simulink model "HydroEye_6DOF_HITL"  (R2024b)
settings: Solver=VariableStepAuto  StartTime=0.0  StopTime=1200  RelTol=1e-3
undefined symbols (not defined in the file): alpha_vec_Cn0, b, b_ref, beta_vec_Cn0, c, CD_flaps, CDo_CD_elev, cg, CL_flaps, Clbeta, Clda, CLo_CL_elev, Clo_Cl_rudder, Clp, Clr, Cm0, Cm_flaps, Cmda, Cmde, Cmo_Cm_elev, Cmq, Cn0, Cnda, Cno_Cn_rudder, Cnp, Cnr, contact, control, cp, CX0, CXda, CXde, CYbeta, CYda, Cyo_Cy_rudder, CZ0, CZda, CZde, d_ref, Earth, F, fractalcoef, Light, m_to_mm, mass, MIL, ms_to_cms, Payload, ref_height, ref_lat, ref_lon, SampleTime, uT_to_gauss, WGS84
libraries: uavmavlinklib x7, simulink_extras x4, aerolibwind2 x3, aerolibatmos2 x2, aerolibasang x2, px4MAVLinkBridgelib x2, shared6dof x1, aerolibadyn x1, simulink x1, aerolibtransform2 x1, sensorgpslib x1, robotcorelib x1
(part 1 of 2)
settings Model: Creator=01  LastModifiedBy=01
settings OptimizationCC: ReuseModelBlockBuffer=off
settings RTWCC: GPUComputeCapability=3.5

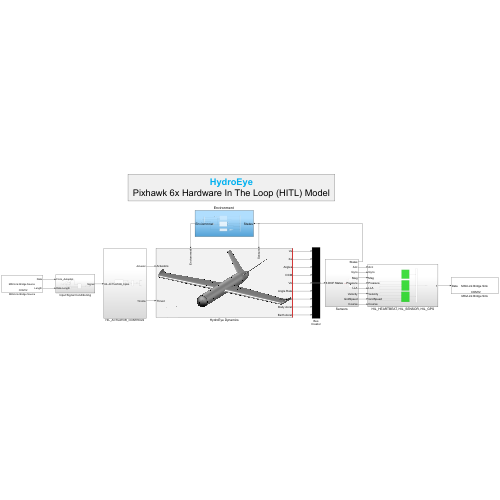
[thumbnail: Simulink's stored preview of the top-level diagram]
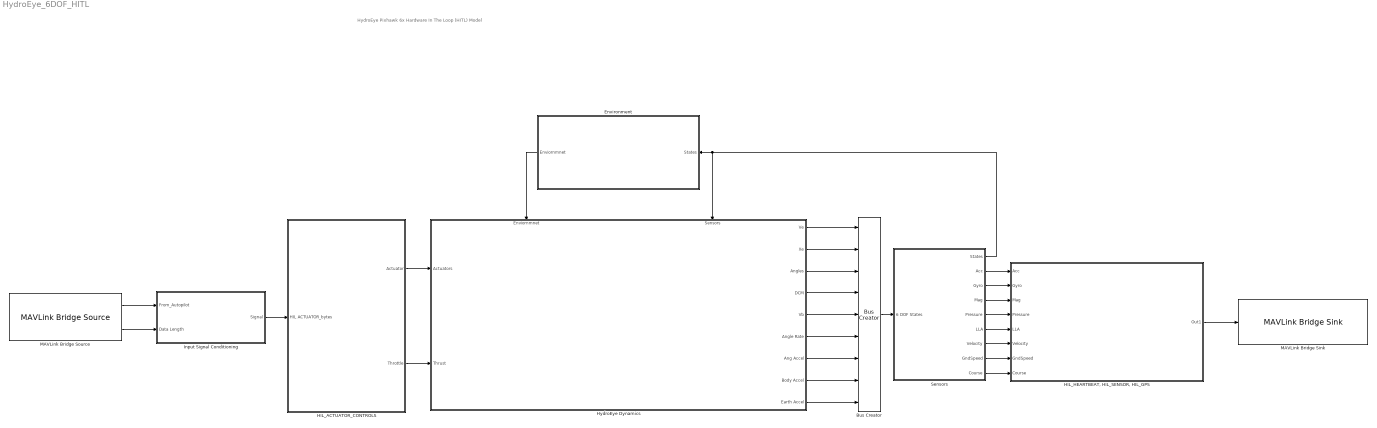
== system HydroEye_6DOF_HITL ==
  note: HydroEye
      | Pixhawk 6x Hardware In The Loop (HITL) Model
  Bus Creator : BusCreator  Inputs=9
  "Environment " : Subsystem
      settings: LibrarySourceBlock=|
      | aeroblk_lib_HL20/HL20
      | Airframe/Environment Models
  HIL_ACTUATOR_CONTROLS : Subsystem
  "HIL_HEARTBEAT, HIL_SENSOR, HIL_GPS" : Subsystem
  HydroEye Dynamics : Subsystem
      settings: PortSchema="{\"entries\":[{\"content\":{\"sides\":[{\"content\":{\"connectorIds\":[\"In1\",\"In2\"]},\"type\":\"ConnectorPlacement.EquallySpacedRectSide\",\"uuid\":\"55fccbc5-ee7f-44af-8150-33bff5380d0a\"},{\"content\":{\"connectorIds\":[\"Out1\",\"Out2\",\"Out3\",\"Out4\",\"Out5\",\"Out6\",\"Out7\",\"Out8\",\"Out9\"],\"side\":\"RIGHT\"},\"type\":\"ConnectorPlacement.EquallySpacedRectSide\",\"uuid\":\"71396e1b-5d20-4c4e-8e08-515b892d20e7\"},{\"content\":{\"connectorIds\":[\"In3\",\"In4\"],\"side\":\"TOP\"},\"type\":\"ConnectorPlacement.EquallySpacedRectSide\",\"uuid\":\"0174f631-e350-4c9f-98c1-67a3807d9144\"}]},\"type\":\"ConnectorPlacement.EquallySpacedConnector\",\"uuid\":\"de3a6adf-aa37-4a7c-9368-465ba59bc2f3\"}],\"packageUris\":[\"http://schema.mathworks.com/mf0/Connector/R2020b\"],\"version\":\"1.0\"}"
      mask Display: image('s.PNG');
  Input Signal Conditioning : Subsystem
  MAVLink Bridge Sink : px4MAVLinkBridgelib/MAVLink Bridge Sink  PixhawkSerialPorttemp=Specify manually  PixhawkSerialPortManually=COM12  FieldTable={ 'UDP', '127.0.0.1', '14550' }
  MAVLink Bridge Source : px4MAVLinkBridgelib/MAVLink Bridge Source  PixhawkSerialPorttemp=Specify manually  PixhawkSerialPortManually=COM12  dataLength=MAVLink_Input_Read_Size  FieldTable={ 'UDP', '127.0.0.1', '14550' }  SampleTime=SampleTime
  Sensors : Subsystem
  wires:
  Sensors/1(States) -> HydroEye Dynamics/4(Sensors), "Environment "/1(States)
  Bus Creator/1 -> Sensors/1(6 DOF States)
  HydroEye Dynamics/2(Xe) -> Bus Creator/2
  "Environment "/1(Enviornmnet) -> HydroEye Dynamics/3(Enviornmnet)
  HydroEye Dynamics/1(Ve) -> Bus Creator/1
  HydroEye Dynamics/3(Angles) -> Bus Creator/3
  HydroEye Dynamics/4(DCM) -> Bus Creator/4
  HydroEye Dynamics/5(Vb) -> Bus Creator/5
  HydroEye Dynamics/6(Angle Rate) -> Bus Creator/6
  HydroEye Dynamics/7(Ang Accel) -> Bus Creator/7
  HydroEye Dynamics/8(Body Accel) -> Bus Creator/8
  HydroEye Dynamics/9(Earth Accel) -> Bus Creator/9
  MAVLink Bridge Source/1 -> Input Signal Conditioning/1(From_Autopilot)
  MAVLink Bridge Source/2 -> Input Signal Conditioning/2(Data Length)
  HIL_ACTUATOR_CONTROLS/1(Actuator) -> HydroEye Dynamics/1(Actuators)
  Sensors/2(Acc) -> "HIL_HEARTBEAT, HIL_SENSOR, HIL_GPS"/1(Acc)
  Sensors/3(Gyro) -> "HIL_HEARTBEAT, HIL_SENSOR, HIL_GPS"/2(Gyro)
  Sensors/4(Mag) -> "HIL_HEARTBEAT, HIL_SENSOR, HIL_GPS"/3(Mag)
  Sensors/5(Pressure) -> "HIL_HEARTBEAT, HIL_SENSOR, HIL_GPS"/4(Pressure)
  Sensors/6(LLA) -> "HIL_HEARTBEAT, HIL_SENSOR, HIL_GPS"/5(LLA)
  Sensors/7(Velocity) -> "HIL_HEARTBEAT, HIL_SENSOR, HIL_GPS"/6(Velocity)
  Sensors/8(GndSpeed) -> "HIL_HEARTBEAT, HIL_SENSOR, HIL_GPS"/7(GndSpeed)
  Sensors/9(Course) -> "HIL_HEARTBEAT, HIL_SENSOR, HIL_GPS"/8(Course)
  "HIL_HEARTBEAT, HIL_SENSOR, HIL_GPS"/1(Out1) -> MAVLink Bridge Sink/1
  Input Signal Conditioning/1(Signal) -> HIL_ACTUATOR_CONTROLS/1(HIL ACTUATOR_bytes)
  HIL_ACTUATOR_CONTROLS/2(Throttle) -> HydroEye Dynamics/2(Thrust)

== system HydroEye_6DOF_HITL/Environment  ==
  States : Inport
  Bus Creator : BusCreator  Inputs=5
  Bus Selector : BusSelector  OutputSignals=Raw States.Ve,Raw States.DCM,LLA
  COESA Atmosphere Model : aerolibatmos2/COESA Atmosphere Model  units=Metric (MKS)  spec=1976 COESA-extended U.S. Standard Atmosphere  model=Profile  profile_var=High temperature  profile_percent=10%  profile_alt=5 km (16404 ft)  envelope_var=High temperature  envelope_percent=1%  action=None
      settings: LibrarySourceBlock=|
      | aeroblk_lib_HL20/HL20
      | Airframe/Environment Models/COESA Atmosphere Model
  Dot Product : DotProduct  Commented=on  SaturateOnIntegerOverflow=on  InputSameDT=off  OutDataTypeStr=Inherit: Inherit via internal rule
  Gravity in Earth Axes : Gain  Gain=[ 0 0 1]  SaturateOnIntegerOverflow=on  OutDataTypeStr=Inherit: Same as input  ParamDataTypeStr=Inherit: Same as input
  Selector : Selector  InputPortWidth=3  IndexOptions=Index vector (dialog)  Indices=3  OutputSizes=1
  Terminator : Terminator
  Terminator1 : Terminator
  V : Math  Commented=on  Operator=sqrt  SignedPower=on
  "WGS84 Gravity Model  " : GravityWGS84  action=None
  Wind : Subsystem  Commented=on
  Enviornmnet : Outport
  wires:
  V/1 -> Wind/1(Airspeed)
  "WGS84 Gravity Model  "/1 -> Gravity in Earth Axes/1
  COESA Atmosphere Model/1 -> Terminator/1
  COESA Atmosphere Model/3 -> Terminator1/1
  COESA Atmosphere Model/2 -> Bus Creator/3
  COESA Atmosphere Model/4 -> Bus Creator/4  "rho"
  Selector/1 -> Wind/2(Altitude), COESA Atmosphere Model/1
  Dot Product/1 -> V/1
  Wind/2(p,q,r wind) -> Bus Creator/2  "p,q,r wind"
  Wind/1(u,v,w wind) -> Bus Creator/1  "u,v,w wind"
  Gravity in Earth Axes/1 -> Bus Creator/5  "gravity acceleration"
  States/1 -> Bus Selector/1
  Bus Selector/2 -> Wind/3(DCM)  "<DCM>"
  Bus Selector/1 -> Dot Product/1, Dot Product/2  "<Ve>"
  Bus Selector/3 -> "WGS84 Gravity Model  "/1, Selector/1  "<LLA>"
  Bus Creator/1 -> Enviornmnet/1  "Environment"

== system HydroEye_6DOF_HITL/HIL_ACTUATOR_CONTROLS ==
  HIL ACTUATOR_bytes : Inport
  Bus Selector : BusSelector  OutputSignals=Payload.controls
  Data Type Conversion : DataTypeConversion  OutDataTypeStr=double  SaturateOnIntegerOverflow=off  RndMeth=Floor
  MAVLink Deserializer : uavmavlinklib/MAVLink Deserializer  dialectSource=Select from standard MAVLink dialects  dialect=common.xml  dialectCustom=common.xml  version=2  messageType=HIL_ACTUATOR_CONTROLS  inputDataLength=off  SystemIDFilter=off  systemID=1  ComponentIDFilter=off  componentID=1  queueMsg=off  queueMsgSize=50  dropNum=off
  Saturation : Saturate  UpperLimit=1  LowerLimit=0
  Selector1 : Selector  InputPortWidth=16  IndexOptions=Index vector (dialog)  Indices=[1:4]  OutputSizes=1
  Terminator : Terminator
  Actuator : Outport
  Throttle : Outport  Port=2
  wires:
  Data Type Conversion/1 -> Selector1/1
  MAVLink Deserializer/1 -> Terminator/1
  MAVLink Deserializer/2 -> Bus Selector/1
  Bus Selector/1 -> Data Type Conversion/1  "<controls>"
  HIL ACTUATOR_bytes/1 -> MAVLink Deserializer/1
  Selector1/1 -> Saturation/1  "Controls"
  Saturation/1 -> Throttle/1, Actuator/1

== system HydroEye_6DOF_HITL/HIL_HEARTBEAT, HIL_SENSOR, HIL_GPS ==
  Acc : Inport
  Gyro : Inport  Port=2
  Mag : Inport  Port=3
  Pressure : Inport  Port=4
  LLA : Inport  Port=5
  Velocity : Inport  Port=6
  GndSpeed : Inport  Port=7
  Course : Inport  Port=8
  HIL_GPS : Subsystem
  HIL_SENSOR : Subsystem
  Mux : Mux  Inputs=3
  Send Heartbeat : Subsystem
  Out1 : Outport
  wires:
  Send Heartbeat/1(HEARTBEAT_bytes) -> Mux/1
  Velocity/1 -> HIL_GPS/2(Velocity)
  HIL_GPS/1(HIL_GPS_bytes) -> Mux/3
  HIL_SENSOR/1(HIL_SENSOR_bytes) -> Mux/2
  GndSpeed/1 -> HIL_GPS/3(GndSpeed)
  LLA/1 -> HIL_GPS/1(LLA)
  Mag/1 -> HIL_SENSOR/3(Mag)
  Mux/1 -> Out1/1
  Pressure/1 -> HIL_SENSOR/4(Pressure)
  Course/1 -> HIL_GPS/4(Course)
  Gyro/1 -> HIL_SENSOR/2(Gyro)
  Acc/1 -> HIL_SENSOR/1(Acc)

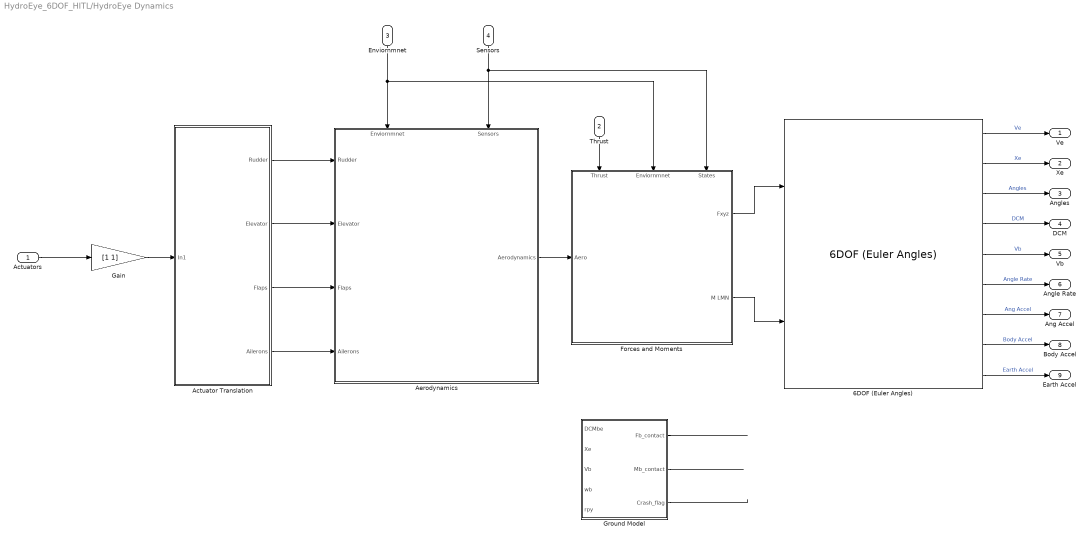
== system HydroEye_6DOF_HITL/HydroEye Dynamics ==
  Actuators : Inport
  Thrust : Inport  Port=2
  Enviornmnet : Inport  Port=3
  Sensors : Inport  Port=4
  6DOF (Euler Angles) : shared6dof/6DOF (Euler Angles)  units=Metric (MKS)  mtype=Fixed  rep=Euler Angles  xme_0=init.pos  Vm_0=init.v  eul_0=init.angles  pm_0=init.angRates  mass_0=mass  mass_e=0.5  mass_f=2.0  inertia=I  inertia_e=eye(3)  inertia_f=2*eye(3)  k_quat=1.0  vre_flag=on  abi_flag=on  aMode=aMode  xme_statename=''  Vm_statename=''  eul_statename=''  quat_statename=''  pm_statename=''  mass_statename=''
      settings: LibrarySourceBlock=|
      | aeroblk_lib_HL20/HL20
      | Airframe/6DOF (Euler Angles)
  Actuator Translation : Subsystem
  Aerodynamics : Subsystem
      settings: PortSchema="{\"entries\":[{\"content\":{\"sides\":[{\"content\":{\"connectorIds\":[\"In1\",\"In2\"]},\"type\":\"ConnectorPlacement.EquallySpacedRectSide\",\"uuid\":\"6872a9e6-04cc-43fe-8307-2d3d33caa71d\"},{\"content\":{\"side\":\"RIGHT\"},\"type\":\"ConnectorPlacement.EquallySpacedRectSide\",\"uuid\":\"de5f8d1c-5c0e-46cb-94c5-3e4cce4cf93c\"},{\"content\":{\"connectorIds\":[\"In3\",\"In4\",\"In5\",\"In6\"],\"side\":\"TOP\"},\"type\":\"ConnectorPlacement.EquallySpacedRectSide\",\"uuid\":\"d9dd98e0-8ff1-4387-90e5-0ec057a718ca\"},{\"content\":{\"connectorIds\":[\"Out1\"],\"side\":\"BOTTOM\"},\"type\":\"ConnectorPlacement.EquallySpacedRectSide\",\"uuid\":\"12421dae-0177-4f1a-9b31-64f8981b692b\"}]},\"type\":\"ConnectorPlacement.EquallySpacedConnector\",\"uuid\":\"9e39648a-6fb6-4479-b0ac-1c0f654141e6\"}],\"packageUris\":[\"http://schema.mathworks.com/mf0/Connector/R2020b\"],\"version\":\"1.0\"}"
  Forces and Moments : Subsystem
      settings: PortSchema="{\"entries\":[{\"content\":{\"sides\":[{\"content\":{\"connectorIds\":[\"In1\"]},\"type\":\"ConnectorPlacement.EquallySpacedRectSide\",\"uuid\":\"3fce203a-ae0b-4bce-a87b-30de4173aaf5\"},{\"content\":{\"connectorIds\":[\"Out1\",\"Out2\"],\"side\":\"RIGHT\"},\"type\":\"ConnectorPlacement.EquallySpacedRectSide\",\"uuid\":\"d2fe57eb-25a4-4a3f-81a0-5ad8de127e30\"},{\"content\":{\"connectorIds\":[\"In2\",\"In3\",\"In4\"],\"side\":\"TOP\"},\"type\":\"ConnectorPlacement.EquallySpacedRectSide\",\"uuid\":\"a48e6f39-78f9-49f0-a87f-61fc55168fed\"}]},\"type\":\"ConnectorPlacement.EquallySpacedConnector\",\"uuid\":\"9bf99150-9e27-4a02-9f3a-86824a85a991\"}],\"packageUris\":[\"http://schema.mathworks.com/mf0/Connector/R2020b\"],\"version\":\"1.0\"}"
      settings: LibrarySourceBlock=|
      | aeroblk_lib_HL20/HL20
      | Airframe/Forces and Moments
  Gain : Gain  Gain=[1 1]
  Ground Model : Subsystem
  Ve : Outport
  Xe : Outport  Port=2
  Angles : Outport  Port=3
  DCM : Outport  Port=4
  Vb : Outport  Port=5
  Angle Rate : Outport  Port=6
  Ang Accel : Outport  Port=7
  Body Accel : Outport  Port=8
  Earth Accel : Outport  Port=9
  wires:
  Forces and Moments/1(Fxyz) -> 6DOF (Euler Angles)/1
  Sensors/1 -> Forces and Moments/4(States), Aerodynamics/2(Sensors)
  Enviornmnet/1 -> Forces and Moments/3(Enviornmnet), Aerodynamics/1(Enviornmnet)
  Forces and Moments/2(M LMN) -> 6DOF (Euler Angles)/2
  Actuators/1 -> Gain/1
  6DOF (Euler Angles)/4 -> DCM/1  "DCM"
  6DOF (Euler Angles)/2 -> Xe/1  "Xe"
  6DOF (Euler Angles)/1 -> Ve/1  "Ve"
  6DOF (Euler Angles)/3 -> Angles/1  "Angles"
  6DOF (Euler Angles)/6 -> Angle Rate/1  "Angle Rate"
  6DOF (Euler Angles)/8 -> Body Accel/1  "Body Accel"
  6DOF (Euler Angles)/5 -> Vb/1  "Vb"
  6DOF (Euler Angles)/9 -> Earth Accel/1  "Earth Accel"
  6DOF (Euler Angles)/7 -> Ang Accel/1  "Ang Accel"
  Thrust/1 -> Forces and Moments/2(Thrust)
  Ground Model/3(Crash_flag) -> ?
  Ground Model/1(Fb_contact) -> ?
  Ground Model/2(Mb_contact) -> ?
  Aerodynamics/1("Aerodynamics ") -> Forces and Moments/1(Aero)
  Gain/1 -> Actuator Translation/1(In1)
  Actuator Translation/1(Rudder) -> Aerodynamics/3(Rudder)
  Actuator Translation/2(Elevator) -> Aerodynamics/4(Elevator)
  Actuator Translation/3(Flaps) -> Aerodynamics/5(Flaps)
  Actuator Translation/4(Ailerons) -> Aerodynamics/6(Ailerons)

== system HydroEye_6DOF_HITL/Input Signal Conditioning ==
  From_Autopilot : Inport
  Data Length : Inport  Port=2
  Constant : Constant
  Constant1 : Constant  Value=0  OutDataTypeStr=uint8  SampleTime=-1
  Data Type Conversion : DataTypeConversion  OutDataTypeStr=double  SaturateOnIntegerOverflow=off  RndMeth=Floor
  Mux1 : Mux  Inputs=2
  Reshape : Reshape
  Selector : Selector  InputPortWidth=MAVLink_Input_Read_Size  IndexOptions=Starting and ending indices (port)  Indices=[1 3]  OutputSizes=1
  Switch : Switch  Criteria=u2 > Threshold  SaturateOnIntegerOverflow=off  InputSameDT=off
  Signal : Outport
  wires:
  Reshape/1 -> Signal/1
  Mux1/1 -> Selector/2
  Data Length/1 -> Data Type Conversion/1
  Constant/1 -> Mux1/1
  Selector/1 -> Switch/1
  From_Autopilot/1 -> Selector/1
  Constant1/1 -> Switch/3
  Switch/1 -> Reshape/1
  Data Type Conversion/1 -> Switch/2, Mux1/2

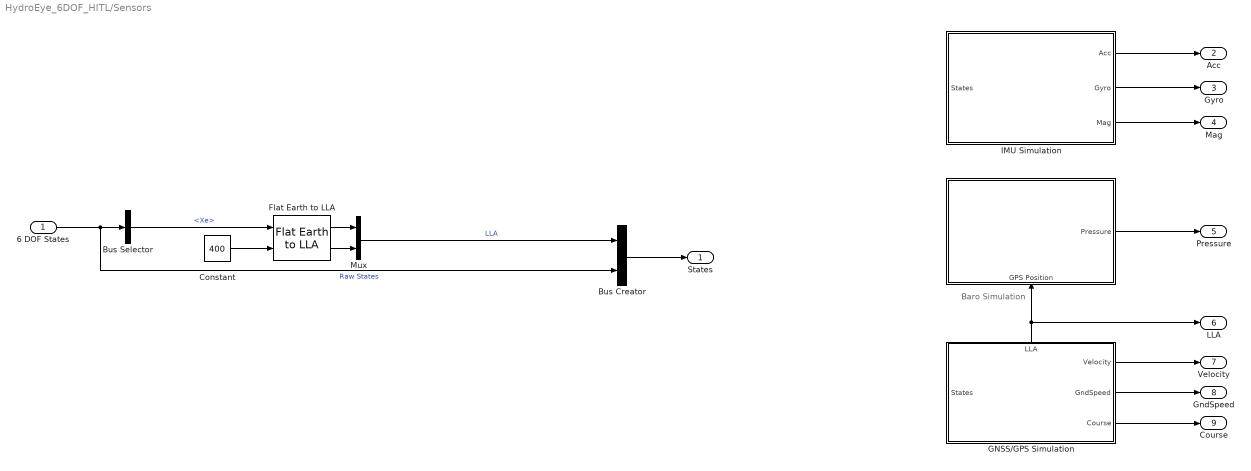
== system HydroEye_6DOF_HITL/Sensors ==
  note: Baro Simulation
  6 DOF States : Inport
  " " : Subsystem
      settings: PortSchema="{\"entries\":[{\"content\":{\"sides\":[{\"content\":{\"connectorIds\":[]},\"type\":\"ConnectorPlacement.EquallySpacedRectSide\",\"uuid\":\"7ecc8b21-8f8f-4144-826a-6b68e30dbf7d\"},{\"content\":{\"connectorIds\":[\"Out1\"],\"side\":\"RIGHT\"},\"type\":\"ConnectorPlacement.EquallySpacedRectSide\",\"uuid\":\"81a1dd55-8330-4386-9921-36c0eb60d526\"},{\"content\":{\"connectorIds\":[],\"side\":\"TOP\"},\"type\":\"ConnectorPlacement.EquallySpacedRectSide\",\"uuid\":\"b99caff5-b40d-407d-b30e-35210c1aee1d\"},{\"content\":{\"connectorIds\":[\"In1\"],\"side\":\"BOTTOM\"},\"type\":\"ConnectorPlacement.EquallySpacedRectSide\",\"uuid\":\"18bfda3d-4fab-4e61-9ebc-e384e51de306\"}]},\"type\":\"ConnectorPlacement.EquallySpacedConnector\",\"uuid\":\"17ab4e96-b761-4c62-a0bb-ab626dac3eaa\"}],\"packageUris\":[\"http://schema.mathworks.com/mf0/Connector/R2020b\"],\"version\":\"1.0\"}"
  Bus Creator : BusCreator  Inputs=2
  Bus Selector : BusSelector  OutputSignals=Xe
  Constant : Constant  Value=400
  Flat Earth to LLA : aerolibtransform2/Flat Earth to LLA  units=Metric (MKS)  ptype=Earth (WGS84)  F=1/298.257223563  R=6378137  refPosPort=off  LL0=[ 24 46 ]  psi=0
  GNSS/GPS Simulation : Subsystem
      settings: PortSchema="{\"entries\":[{\"content\":{\"sides\":[{\"content\":{\"connectorIds\":[\"In1\"]},\"type\":\"ConnectorPlacement.EquallySpacedRectSide\",\"uuid\":\"4934e8ff-5d4b-4e11-968d-c23bd62383a0\"},{\"content\":{\"connectorIds\":[\"Out1\",\"Out2\",\"Out3\"],\"side\":\"RIGHT\"},\"type\":\"ConnectorPlacement.EquallySpacedRectSide\",\"uuid\":\"9ec8bc0a-2d3c-4dca-835c-010ac29b6ebc\"},{\"content\":{\"connectorIds\":[\"Out4\"],\"side\":\"TOP\"},\"type\":\"ConnectorPlacement.EquallySpacedRectSide\",\"uuid\":\"04f09eb4-1bd9-450e-b951-47054bdd92ad\"}]},\"type\":\"ConnectorPlacement.EquallySpacedConnector\",\"uuid\":\"9a5920cf-a58d-4c98-839b-fbac94edbe7e\"}],\"packageUris\":[\"http://schema.mathworks.com/mf0/Connector/R2020b\"],\"version\":\"1.0\"}"
  IMU Simulation : Subsystem
  Mux : Mux  Inputs=2
  States : Outport
  Acc : Outport  Port=2
  Gyro : Outport  Port=3
  Mag : Outport  Port=4
  Pressure : Outport  Port=5
  LLA : Outport  Port=6
  Velocity : Outport  Port=7
  GndSpeed : Outport  Port=8
  Course : Outport  Port=9
  wires:
  6 DOF States/1 -> Bus Creator/2, Bus Selector/1  "Raw States"
  Bus Selector/1 -> Flat Earth to LLA/1  "<Xe>"
  Flat Earth to LLA/2 -> Mux/2
  Flat Earth to LLA/1 -> Mux/1
  Mux/1 -> Bus Creator/1  "LLA"
  Bus Creator/1 -> States/1
  Constant/1 -> Flat Earth to LLA/2
  GNSS/GPS Simulation/1(Velocity) -> Velocity/1
  " "/1(Pressure) -> Pressure/1
  ? -> IMU Simulation/1(States), GNSS/GPS Simulation/1(States)
  IMU Simulation/3(Mag) -> Mag/1
  GNSS/GPS Simulation/3(Course) -> Course/1
  GNSS/GPS Simulation/2(GndSpeed) -> GndSpeed/1
  GNSS/GPS Simulation/4(LLA) -> LLA/1, " "/1(GPS Position)
  IMU Simulation/2(Gyro) -> Gyro/1
  IMU Simulation/1(Acc) -> Acc/1

== system HydroEye_6DOF_HITL/Environment /Wind ==
  Airspeed : Inport  Unit=m/s
  Altitude : Inport  Port=2  Unit=m
  DCM : Inport  Port=3
  Discrete Wind Gust Model - On : aerolibwind2/Discrete Wind Gust Model  units=Metric (MKS)  Gx=on  Gy=on  Gz=on  t_0=20  d_m=[120 120 80]  v_m=[3.5 3.0 3.0]
      settings: LibrarySourceBlock=|
      | aeroblk_lib_HL20/HL20
      | Airframe/Environment Models/Wind Models/Discrete Wind Gust Model - On
  Dryden Wind Turbulence Model (Continuous (+q -r)) : aerolibwind2/Dryden Wind Turbulence Model  (Continuous (+q -r))  units=Metric (MKS)  spec=MIL-F-8785C  model=Continuous Dryden (+q -r)  W20=5  Wdeg=0  TurbProb=10^-2 - Light  L_high=533.4  Wingspan=4  ts=0.1  Seed=[23341 23342 23343 23344]  T_on=on
      settings: LibrarySourceBlock=|
      | aeroblk_lib_HL20/HL20
      | Airframe/Environment Models/Wind Models/Dryden Wind Turbulence Model
      | (Continuous (+q -r))
  Sum : Sum  Inputs=+++  InputSameDT=on  SaturateOnIntegerOverflow=on  OutDataTypeStr=Inherit: Same as first input
  Wind Shear Model : aerolibwind2/Wind Shear Model  units=Metric (MKS)  phase=Category C - Terminal Flight Phase  W_20=1  Wdeg=0
      settings: LibrarySourceBlock=|
      | aeroblk_lib_HL20/HL20
      | Airframe/Environment Models/Wind Models/Wind Shear Model
  u,v,w wind : Outport  Unit=m/s  VectorParamsAs1DForOutWhenUnconnected=off
  p,q,r wind : Outport  Port=2  Unit=rad/s  VectorParamsAs1DForOutWhenUnconnected=off
  wires:
  Altitude/1 -> Wind Shear Model/1, Dryden Wind Turbulence Model (Continuous (+q -r))/1
  Dryden Wind Turbulence Model (Continuous (+q -r))/2 -> p,q,r wind/1
  Airspeed/1 -> Discrete Wind Gust Model - On/1, Dryden Wind Turbulence Model (Continuous (+q -r))/2
  DCM/1 -> Wind Shear Model/2, Dryden Wind Turbulence Model (Continuous (+q -r))/3
  Sum/1 -> u,v,w wind/1
  Discrete Wind Gust Model - On/1 -> Sum/3
  Dryden Wind Turbulence Model (Continuous (+q -r))/1 -> Sum/2
  Wind Shear Model/1 -> Sum/1

== system HydroEye_6DOF_HITL/HIL_HEARTBEAT, HIL_SENSOR, HIL_GPS/HIL_GPS ==
  LLA : Inport
  Velocity : Inport  Port=2
  GndSpeed : Inport  Port=3
  Course : Inport  Port=4
  HIL_GPS Subsystem : Subsystem
  MAVLink Serializer3 : uavmavlinklib/MAVLink Serializer  dialectSource=Select from standard MAVLink dialects  dialect=common.xml  dialectCustom=common.xml  version=2  messageType=HIL_GPS
  Rate Transition : RateTransition  OutPortSampleTime=SampleTime
  Terminator2 : Terminator
  HIL_GPS_bytes : Outport
  wires:
  HIL_GPS Subsystem/1(Out1) -> Rate Transition/1
  Course/1 -> HIL_GPS Subsystem/4(Course)
  MAVLink Serializer3/2 -> Terminator2/1
  LLA/1 -> HIL_GPS Subsystem/1(LLA)
  GndSpeed/1 -> HIL_GPS Subsystem/3(GndSpeed)
  MAVLink Serializer3/1 -> HIL_GPS_bytes/1
  Velocity/1 -> HIL_GPS Subsystem/2(Velocity)
  Rate Transition/1 -> MAVLink Serializer3/1

== system HydroEye_6DOF_HITL/HIL_HEARTBEAT, HIL_SENSOR, HIL_GPS/HIL_SENSOR ==
  Acc : Inport
  Gyro : Inport  Port=2
  Mag : Inport  Port=3
  Pressure : Inport  Port=4
  HIL_SENSOR Creation subsystem : Subsystem
  MAVLink Serializer1 : uavmavlinklib/MAVLink Serializer  dialectSource=Select from standard MAVLink dialects  dialect=common.xml  dialectCustom=common.xml  version=2  messageType=HIL_SENSOR
  Rate Transition : RateTransition  OutPortSampleTime=SampleTime
  Terminator : Terminator
  HIL_SENSOR_bytes : Outport
  wires:
  Pressure/1 -> HIL_SENSOR Creation subsystem/4(Pressure)
  Acc/1 -> HIL_SENSOR Creation subsystem/1(Acc)
  MAVLink Serializer1/2 -> Terminator/1
  MAVLink Serializer1/1 -> HIL_SENSOR_bytes/1
  Mag/1 -> HIL_SENSOR Creation subsystem/3(Mag)
  HIL_SENSOR Creation subsystem/1(HIL Sensor) -> Rate Transition/1
  Gyro/1 -> HIL_SENSOR Creation subsystem/2(Gyro)
  Rate Transition/1 -> MAVLink Serializer1/1

== system HydroEye_6DOF_HITL/HIL_HEARTBEAT, HIL_SENSOR, HIL_GPS/Send Heartbeat ==
  Bus Assignment : BusAssignment  AssignedSignals=Payload.autopilot,Payload.type
  Constant : Constant  SampleTime=-1
  Constant1 : Constant  Value=12  SampleTime=-1
  Data Type Conversion : DataTypeConversion  OutDataTypeStr=uint8  SaturateOnIntegerOverflow=off  RndMeth=Floor
  Data Type Conversion1 : DataTypeConversion  OutDataTypeStr=uint8  SaturateOnIntegerOverflow=off  RndMeth=Floor
  MAVLink Blank Message : uavmavlinklib/MAVLink Blank Message  dialectSource=Select from standard MAVLink dialects  dialect=common.xml  dialectCustom=common.xml  version=2  messageType=HEARTBEAT  SystemID=2  ComponentID=51  SampleTime=SampleTime
  MAVLink Serializer : uavmavlinklib/MAVLink Serializer  dialectSource=Select from standard MAVLink dialects  dialect=common.xml  dialectCustom=common.xml  version=2  messageType=HEARTBEAT
  Terminator4 : Terminator
  HEARTBEAT_bytes : Outport
  wires:
  Bus Assignment/1 -> MAVLink Serializer/1
  Constant/1 -> Data Type Conversion/1
  MAVLink Serializer/1 -> HEARTBEAT_bytes/1
  Data Type Conversion1/1 -> Bus Assignment/3
  Data Type Conversion/1 -> Bus Assignment/2
  MAVLink Serializer/2 -> Terminator4/1
  Constant1/1 -> Data Type Conversion1/1
  MAVLink Blank Message/1 -> Bus Assignment/1

== system HydroEye_6DOF_HITL/HydroEye Dynamics/Actuator Translation ==
  note: https://ardupilot.org/plane/docs/guide-vtail-plane.html#guide-vtail-plane
      |
      | Basically reversed ArduPilot's V-tail mixing, to translate to an elevator & rudder config, making us need less data.
      |
      | So the rudder commads in deg for each ruddervator is mixed as a percentage of elevator adn rudder deflection.
      |
      | The gain is a mixing percantage and it is IMPORTANT to update it when changing it in the parameters OR ELSE the translation will be wrong
  In1 : Inport
  Demux : Demux
  Gain : Gain  Gain=0.5
  Gain1 : Gain  Gain=0.5
  Sum : Sum  Inputs=|-+
  Sum1 : Sum  Inputs=|++
  Rudder : Outport
  Elevator : Outport  Port=2
  Flaps : Outport  Port=3
  Ailerons : Outport  Port=4
  wires:
  In1/1 -> Demux/1
  Demux/1 -> Gain/1  "Ruddervator Right"
  Demux/2 -> Gain1/1  "Ruddervator Left"
  Sum/1 -> Rudder/1
  Sum1/1 -> Elevator/1
  Gain/1 -> Sum1/1, Sum/1
  Gain1/1 -> Sum1/2, Sum/2
  Demux/3 -> Flaps/1  "Flaps"
  Demux/4 -> Ailerons/1  "Ailerons"

== system HydroEye_6DOF_HITL/HydroEye Dynamics/Aerodynamics ==
  note: Order is for stability input in aero forces block
  Enviornmnet : Inport
  Sensors : Inport  Port=2
  Rudder : Inport  Port=3
  Elevator : Inport  Port=4
  Flaps : Inport  Port=5
  Ailerons : Inport  Port=6
  Aero Coeff : Subsystem
  Aerodynamic Coefficients : Subsystem  Commented=on
      settings: LibrarySourceBlock=|
      | aeroblk_lib_HL20/HL20
      | Airframe/Aerodynamic
      | Coefficients
  Alpha,Beta,q : Subsystem
      settings: LibrarySourceBlock=|
      | aeroblk_lib_HL20/HL20
      | Airframe/Alpha,Beta,Mach
  Bus Creator : BusCreator  Inputs=2
  Demux : Demux  Outputs=2
  Mux : Mux  Inputs=6
  Radians to Degrees : simulink_extras/Transformations/Radians to Degrees
  Radians to Degrees1 : simulink_extras/Transformations/Radians to Degrees
  "Aerodynamics " : Outport
  wires:
  Sensors/1 -> Aero Coeff/7(Sensors), Alpha,Beta,q/2(Sensors)
  Enviornmnet/1 -> Alpha,Beta,q/1(Enviornmnet)
  Alpha,Beta,q/2(qbar) -> Bus Creator/2  "qbar"
  Mux/1 -> Bus Creator/1  "Aero Coeff"
  Alpha,Beta,q/1(Incid) -> Demux/1
  Aero Coeff/1(CD) -> Mux/1  "CD"
  Aero Coeff/2(CY) -> Mux/2  "CY"
  Aero Coeff/3(CL) -> Mux/3  "CL"
  Aero Coeff/4(Cl) -> Mux/4  "Cl"
  Aero Coeff/5(Cm) -> Mux/5  "Cm"
  Aero Coeff/6(Cn) -> Mux/6  "Cn"
  Radians to Degrees/1 -> Aero Coeff/1(Alpha)  "alpha"
  Radians to Degrees1/1 -> Aero Coeff/2(Beta)  "beta"
  Demux/2 -> Radians to Degrees1/1
  Demux/1 -> Radians to Degrees/1  "a rad"
  Bus Creator/1 -> "Aerodynamics "/1
  Rudder/1 -> Aero Coeff/3(Rudder)
  Elevator/1 -> Aero Coeff/4(Elevator)
  Flaps/1 -> Aero Coeff/5(Flaps)
  Ailerons/1 -> Aero Coeff/6(Ailerons)

== system HydroEye_6DOF_HITL/HydroEye Dynamics/Forces and Moments ==
  Aero : Inport
  Thrust : Inport  Port=2
  Enviornmnet : Inport  Port=3
  States : Inport  Port=4
  Aerodynamic Forces and Moments : aerolibadyn/Aerodynamic Forces and Moments   inputAxes=Stability  outputForceAxes=Body  outputMomentAxes=Body  S=Sref  b=b  cbar=c
      settings: LibrarySourceBlock=|
      | aeroblk_lib_HL20/HL20
      | Airframe/Forces and Moments/Aerodynamic
      | Forces and Moments
  Bus Selector : BusSelector  OutputSignals=gravity acceleration
  Bus Selector1 : BusSelector  OutputSignals=Raw States.DCM,Raw States.Vb
  Bus Selector2 : BusSelector  OutputSignals=Aero Coeff,qbar
  Gain1 : Gain  Gain=mass
  Matrix Multiply : Product  Multiplication=Matrix(*)
  Sum : Sum  Inputs=+++  InputSameDT=on  SaturateOnIntegerOverflow=on  OutDataTypeStr=Inherit: Same as first input
  center of gravity : Constant  Value=cg
  center of pressure : Constant  Value=cp
  Fxyz : Outport
  M LMN : Outport  Port=2
  wires:
  Sum/1 -> Fxyz/1
  center of gravity/1 -> Aerodynamic Forces and Moments/3
  center of pressure/1 -> Aerodynamic Forces and Moments/4
  Enviornmnet/1 -> Bus Selector/1
  States/1 -> Bus Selector1/1
  Matrix Multiply/1 -> Sum/3
  Bus Selector/1 -> Gain1/1  "<gravity acceleration>"
  Gain1/1 -> Matrix Multiply/2
  Bus Selector1/1 -> Matrix Multiply/1  "<DCM>"
  Thrust/1 -> Sum/1
  Aerodynamic Forces and Moments/1 -> Sum/2  "Faero"
  Aerodynamic Forces and Moments/2 -> M LMN/1
  Bus Selector1/2 -> Aerodynamic Forces and Moments/5  "<Vb>"
  Aero/1 -> Bus Selector2/1
  Bus Selector2/1 -> Aerodynamic Forces and Moments/1  "<Aero Coeff>"
  Bus Selector2/2 -> Aerodynamic Forces and Moments/2  "<qbar>"

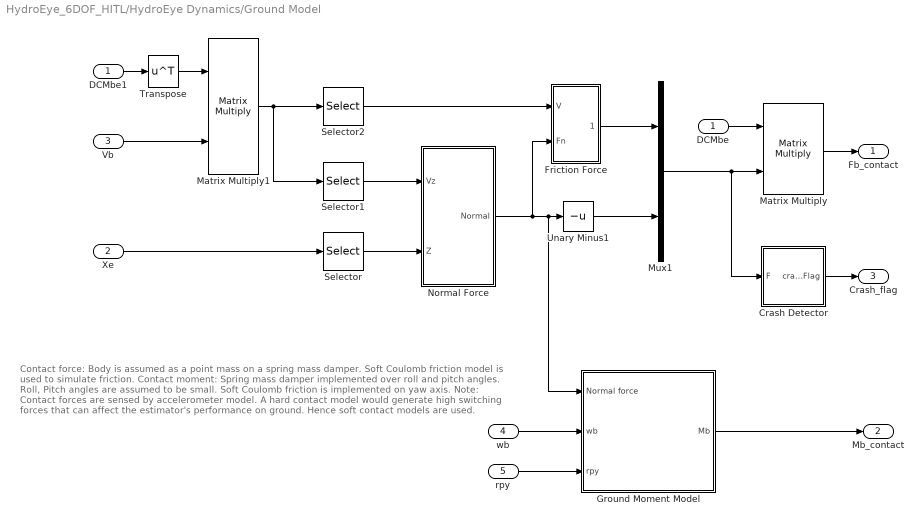
== system HydroEye_6DOF_HITL/HydroEye Dynamics/Ground Model ==
  note: Contact force:
      | Body is assumed as a point mass on a spring mass damper. Soft Coulomb friction model is used to simulate friction.
      |
      | Contact moment:
      | Spring mass damper implemented over roll and pitch angles. Roll, Pitch angles are assumed to be small.
      | Soft Coulomb friction is implemented on yaw axis.
      |
      | Note:
      | Contact forces are sensed by accelerometer model. A hard contact model would generate high switching forces that can affect the estimator's performance on ground. Hence soft contact models are used.
  DCMbe : Inport
  Xe : Inport  Port=2
  Vb : Inport  Port=3
  wb : Inport  Port=4
  rpy : Inport  Port=5
  Crash Detector : Subsystem
  DCMbe1 : InportShadow
  Friction Force : Subsystem
  Ground Moment Model : Subsystem
  Matrix Multiply : Product  Multiplication=Matrix(*)
  Matrix Multiply1 : Product  Multiplication=Matrix(*)
  Mux1 : Mux  Inputs=2
  Normal Force : Subsystem
  Selector : Selector  InputPortWidth=3  IndexOptions=Index vector (dialog)  Indices=[3]  OutputSizes=1
  Selector1 : Selector  InputPortWidth=3  IndexOptions=Index vector (dialog)  Indices=[3]  OutputSizes=1
  Selector2 : Selector  InputPortWidth=3  IndexOptions=Index vector (dialog)  Indices=[1,2]  OutputSizes=1
  Transpose : Math  Operator=transpose
  Unary Minus1 : UnaryMinus
  Fb_contact : Outport
  Mb_contact : Outport  Port=2
  Crash_flag : Outport  Port=3
  wires:
  Crash Detector/1(crashFlag) -> Crash_flag/1
  Xe/1 -> Selector/1
  Selector1/1 -> Normal Force/1(Vz)
  Selector/1 -> Normal Force/2(Z)
  DCMbe/1 -> Matrix Multiply/1
  Matrix Multiply/1 -> Fb_contact/1
  Normal Force/1(Normal) -> Ground Moment Model/1(Normal force), Unary Minus1/1, Friction Force/2(Fn)
  Mux1/1 -> Crash Detector/1(F), Matrix Multiply/2
  Unary Minus1/1 -> Mux1/2
  Selector2/1 -> Friction Force/1(V)
  Friction Force/1(Friction) -> Mux1/1
  DCMbe1/1 -> Transpose/1
  Transpose/1 -> Matrix Multiply1/1
  Vb/1 -> Matrix Multiply1/2
  Matrix Multiply1/1 -> Selector1/1, Selector2/1
  wb/1 -> Ground Moment Model/2(wb)
  rpy/1 -> Ground Moment Model/3(rpy)
  Ground Moment Model/1(Mb) -> Mb_contact/1

== system HydroEye_6DOF_HITL/Sensors/  ==
  GPS Position : Inport
  Extract Altitude : Selector  InputPortWidth=3  IndexOptions=Index vector (dialog)  Indices=[3]  OutputSizes=1
  Gain1 : Gain  Gain=1/m_to_mm
  Gain2 : Gain  Gain=m_to_mm
  Lapse Rate Model : aerolibatmos2/ISA Atmosphere Model  useExtended=off  action=Warning  custom=on  viscosityOut=off  g=9.80665  gamma=1.4  R=287.0531  L=0.0065  h_trop=11000  h_strat=20000  rho0=1.225  P0=101325  T0=288.15  h0=0  S=110.4  Tref=273.15  muref=1.716e-5
  Random Number1 : RandomNumber  Variance=10000  Seed=10  SampleTime=SampleTime
  Sum1 : Sum  Inputs=|++
  Terminator : Terminator
  Terminator1 : Terminator
  Terminator2 : Terminator
  Pressure : Outport
  wires:
  Lapse Rate Model/2 -> Terminator1/1
  Lapse Rate Model/4 -> Terminator2/1
  Lapse Rate Model/1 -> Terminator/1
  Lapse Rate Model/3 -> Pressure/1
  Sum1/1 -> Gain1/1
  Gain2/1 -> Sum1/1
  Extract Altitude/1 -> Gain2/1
  Gain1/1 -> Lapse Rate Model/1
  GPS Position/1 -> Extract Altitude/1
  Random Number1/1 -> Sum1/2  "Pressure_noise"

== system HydroEye_6DOF_HITL/Sensors/GNSS//GPS Simulation ==
  States : Inport
  Bus Selector : BusSelector  OutputSignals=dx,dy,dz  OutputAsBus=on
  Bus Selector1 : BusSelector  OutputSignals=X,Y,Z  OutputAsBus=on
  GPS : sensorgpslib/GPS  DispRefFrame=NED  PositionInputFormat=Local  ReferenceLocation=[ref_lat ref_lon ref_height]  HorizontalPositionAccuracy=0.01  VerticalPositionAccuracy=0.01  VelocityAccuracy=0.01  DecayFactor=0.99  SeedDouble=67  SimulateUsing=Interpreted execution
  Reshape1 : Reshape  OutputDimensionality=Row vector (2-D)
  Reshape3 : Reshape  OutputDimensionality=Row vector (2-D)
  Velocity : Outport
  GndSpeed : Outport  Port=2
  Course : Outport  Port=3
  LLA : Outport  Port=4
  wires:
  Reshape3/1 -> GPS/1
  GPS/1 -> LLA/1  "lla"
  Bus Selector1/1 -> Reshape3/1
  Bus Selector/1 -> Reshape1/1
  Reshape1/1 -> GPS/2
  GPS/2 -> Velocity/1
  States/1 -> Bus Selector/1, Bus Selector1/1
  GPS/3 -> GndSpeed/1
  GPS/4 -> Course/1

== system HydroEye_6DOF_HITL/Sensors/IMU Simulation ==
  note: Note:
      | we need specific force (accelerometer output) in A-G form, but block gives G-A.
  States : Inport
  Bus Selector1 : BusSelector  OutputSignals=p,q,r  OutputAsBus=on
  Bus Selector2 : BusSelector  OutputSignals=yaw,pitch,roll  OutputAsBus=on
  Bus Selector3 : BusSelector  OutputSignals=ddx,ddy,ddz  OutputAsBus=on
  Coordinate Transformation Conversion1 : robotcorelib/Coordinate Transformation Conversion  InputRepresentation=Euler Angles  InputEulerSequence=ZYX  ShowTrVecInputPort=on  OutputRepresentation=Quaternion  OutputEulerSequence=ZYX  ShowTrVecOutputPort=on  SimulateUsing=Interpreted execution
  Gain : Gain  Gain=-1
  IMU1 : mspsensorlib/IMU  DispRefFrame=NED  TemperaturePort=off  Temperature=25  MagneticFieldPort=off  MagneticFieldNED=[21.5 1.16 43.1]  MagneticFieldENU=[ -2.4169, 27.5550, 16.0849 ]  SeedDouble=87254  SimulateUsing=Interpreted execution  AccelParamsMeasurementRange=Inf  AccelParamsResolution=0  AccelParamsConstantBias=[ 0, 0, 0 ]  AccelParamsAxesMisalignment=[ 0, 0, 0 ]  AccelParamsNoiseDensity=0.0003  AccelParamsBiasInstability=[ 0, 0, 0 ]  AccelParamsBiasInstabilityNumerator=fractalcoef().Numerator  AccelParamsBiasInstabilityDenominator=fractalcoef().Denominator  AccelParamsRandomWalk=[ 0, 0, 0 ]  AccelParamsNoiseType=double-sided  AccelParamsTemperatureBias=[ 0, 0, 0 ]  AccelParamsTemperatureScaleFactor=[ 0, 0, 0 ]  GyroParamsMeasurementRange=Inf  GyroParamsResolution=0  GyroParamsConstantBias=[ 0, 0, 0 ]  GyroParamsAxesMisalignment=[ 0, 0, 0 ]  GyroParamsAccelerationBias=0.0001  GyroParamsNoiseDensity=0.01  GyroParamsBiasInstability=[ 0, 0, 0 ]  GyroParamsBiasInstabilityNumerator=fractalcoef().Numerator  GyroParamsBiasInstabilityDenominator=fractalcoef().Denominator  GyroParamsRandomWalk=[ 0, 0, 0 ]  GyroParamsNoiseType=double-sided  GyroParamsTemperatureBias=[ 0, 0, 0 ]  GyroParamsTemperatureScaleFactor=[ 0, 0, 0 ]  MagParamsMeasurementRange=Inf  MagParamsResolution=0  MagParamsConstantBias=[ 0, 0, 0 ]  MagParamsAxesMisalignment=[ 0, 0, 0 ]  MagParamsNoiseDensity=0.0005  MagParamsBiasInstability=[ 0, 0, 0 ]  MagParamsBiasInstabilityNumerator=fractalcoef().Numerator  MagParamsBiasInstabilityDenominator=fractalcoef().Denominator  MagParamsRandomWalk=[ 0, 0, 0 ]  MagParamsNoiseType=double-sided  MagParamsTemperatureBias=[ 0, 0, 0 ]  MagParamsTemperatureScaleFactor=[ 0, 0, 0 ]
  Reshape : Reshape  OutputDimensionality=Row vector (2-D)
  Reshape2 : Reshape  OutputDimensionality=Row vector (2-D)
  Reshape3 : Reshape  OutputDimensionality=Row vector (2-D)
  Acc : Outport
  Gyro : Outport  Port=2
  Mag : Outport  Port=3
  wires:
  Coordinate Transformation Conversion1/1 -> Reshape3/1
  Reshape3/1 -> IMU1/3
  IMU1/3 -> Mag/1
  IMU1/2 -> Gyro/1
  Reshape/1 -> IMU1/1
  Bus Selector3/1 -> Reshape/1
  IMU1/1 -> Gain/1
  Bus Selector1/1 -> Reshape2/1
  Bus Selector2/1 -> Coordinate Transformation Conversion1/1
  Reshape2/1 -> IMU1/2
  States/1 -> Bus Selector1/1, Bus Selector2/1, Bus Selector3/1
  Gain/1 -> Acc/1  "acc"

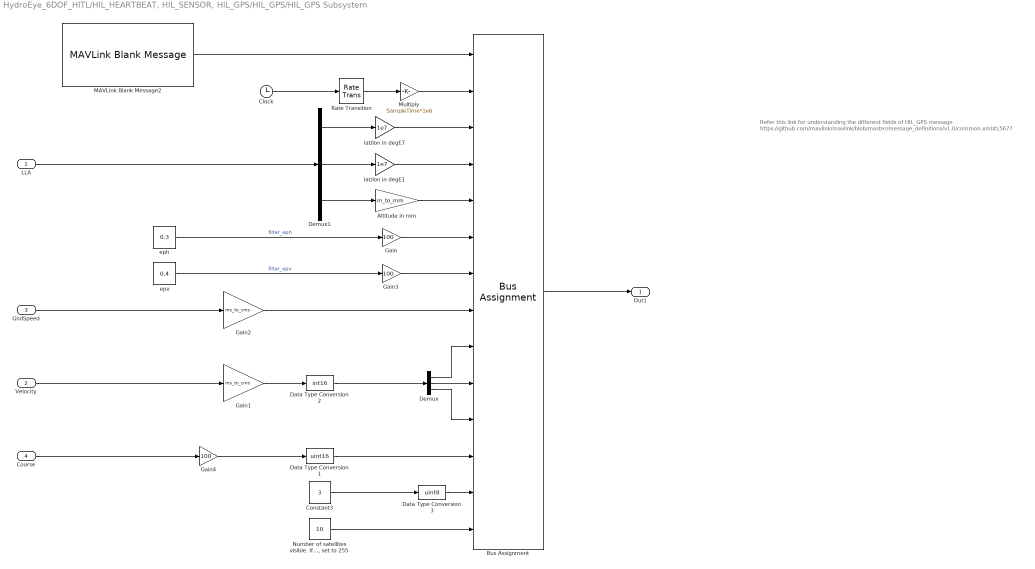
== system HydroEye_6DOF_HITL/HIL_HEARTBEAT, HIL_SENSOR, HIL_GPS/HIL_GPS/HIL_GPS Subsystem ==
  note: Refer this link for understanding the different fields of HIL_GPS message https://github.com/mavlink/mavlink/blob/master/message_definitions/v1.0/common.xml#L5677
  LLA : Inport
  Velocity : Inport  Port=2
  GndSpeed : Inport  Port=3
  Course : Inport  Port=4
  Altitude in mm : Gain  Gain=m_to_mm  OutDataTypeStr=Inherit: Inherit via back propagation
  Bus Assignment : BusAssignment  AssignedSignals=Payload.time_usec,Payload.lat,Payload.lon,Payload.alt,Payload.eph,Payload.epv,Payload.vel,Payload.vn,Payload.ve,Payload.vd,Payload.cog,Payload.fix_type,Payload.satellites_visible
  Clock : Clock
  Constant3 : Constant  Value=3  OutDataTypeStr=Inherit: Inherit via back propagation  SampleTime=-1
  Data Type Conversion1 : DataTypeConversion  OutDataTypeStr=uint16  SaturateOnIntegerOverflow=off  RndMeth=Floor
  Data Type Conversion2 : DataTypeConversion  OutDataTypeStr=int16  SaturateOnIntegerOverflow=off  RndMeth=Floor
  Data Type Conversion3 : DataTypeConversion  OutDataTypeStr=uint8  SaturateOnIntegerOverflow=off  RndMeth=Floor
  Demux : Demux  Outputs=3
  Demux1 : Demux  Outputs=3
  Gain : Gain  Gain=100  OutDataTypeStr=Inherit: Inherit via back propagation
  Gain1 : Gain  Gain=ms_to_cms
  Gain2 : Gain  Gain=ms_to_cms  OutDataTypeStr=uint16
  Gain3 : Gain  Gain=100  OutDataTypeStr=Inherit: Inherit via back propagation
  Gain4 : Gain  Gain=100
  MAVLink Blank Message2 : uavmavlinklib/MAVLink Blank Message  dialectSource=Select from standard MAVLink dialects  dialect=common.xml  dialectCustom=common.xml  version=2  messageType=HIL_GPS  SystemID=2  ComponentID=51  SampleTime=SampleTime
  Multiply : Gain  Gain=SampleTime*1e6  OutDataTypeStr=Inherit: Inherit via back propagation
  "Number of satellites visible. If unknown, set to 255" : Constant  Value=10  OutDataTypeStr=Inherit: Inherit via back propagation  SampleTime=-1
  Rate Transition : RateTransition
  eph : Constant  Value=0.3  SampleTime=-1
  epv : Constant  Value=0.4  SampleTime=-1
  lat/lon in degE1 : Gain  Gain=1e7  OutDataTypeStr=Inherit: Inherit via back propagation
  lat/lon in degE7 : Gain  Gain=1e7  OutDataTypeStr=Inherit: Inherit via back propagation
  Out1 : Outport
  wires:
  Gain2/1 -> Bus Assignment/8
  lat/lon in degE7/1 -> Bus Assignment/3
  Demux1/1 -> lat/lon in degE7/1
  Demux/3 -> Bus Assignment/11
  MAVLink Blank Message2/1 -> Bus Assignment/1
  Gain1/1 -> Data Type Conversion2/1
  Demux1/3 -> Altitude in mm/1
  Demux1/2 -> lat/lon in degE1/1
  Demux/1 -> Bus Assignment/9
  lat/lon in degE1/1 -> Bus Assignment/4
  Altitude in mm/1 -> Bus Assignment/5
  Data Type Conversion2/1 -> Demux/1
  Demux/2 -> Bus Assignment/10
  Bus Assignment/1 -> Out1/1
  "Number of satellites visible. If unknown, set to 255"/1 -> Bus Assignment/14
  Gain/1 -> Bus Assignment/6
  Gain3/1 -> Bus Assignment/7
  LLA/1 -> Demux1/1
  GndSpeed/1 -> Gain2/1
  Velocity/1 -> Gain1/1
  Course/1 -> Gain4/1
  Data Type Conversion1/1 -> Bus Assignment/12
  eph/1 -> Gain/1  "filter_eph"
  epv/1 -> Gain3/1  "filter_epv"
  Data Type Conversion3/1 -> Bus Assignment/13
  Gain4/1 -> Data Type Conversion1/1
  Constant3/1 -> Data Type Conversion3/1
  Clock/1 -> Rate Transition/1
  Rate Transition/1 -> Multiply/1
  Multiply/1 -> Bus Assignment/2

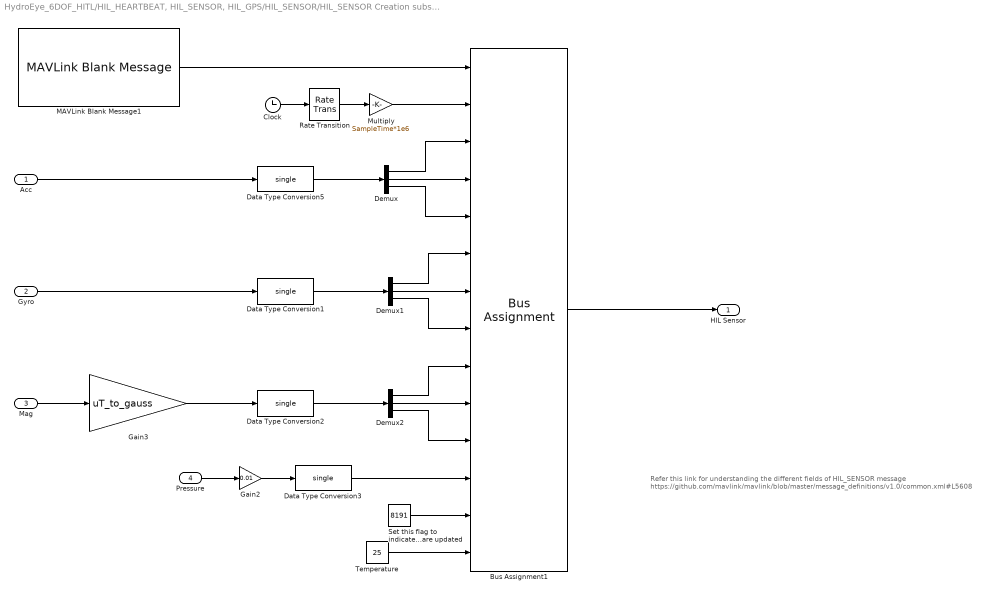
== system HydroEye_6DOF_HITL/HIL_HEARTBEAT, HIL_SENSOR, HIL_GPS/HIL_SENSOR/HIL_SENSOR Creation subsystem ==
  note: Refer this link for understanding the different fields of HIL_SENSOR message https://github.com/mavlink/mavlink/blob/master/message_definitions/v1.0/common.xml#L5608
  Acc : Inport
  Gyro : Inport  Port=2
  Mag : Inport  Port=3
  Pressure : Inport  Port=4
  Bus Assignment1 : BusAssignment  AssignedSignals=Payload.time_usec,Payload.xacc,Payload.yacc,Payload.zacc,Payload.xgyro,Payload.ygyro,Payload.zgyro,Payload.xmag,Payload.ymag,Payload.zmag,Payload.abs_pressure,Payload.fields_updated,Payload.temperature
  Clock : Clock
  Data Type Conversion{1..3,5} (4 alike) : DataTypeConversion  OutDataTypeStr=single  SaturateOnIntegerOverflow=off  RndMeth=Floor
  Demux : Demux  Outputs=3
  Demux1 : Demux  Outputs=3
  Demux2 : Demux  Outputs=3
  Gain2 : Gain  Gain=0.01  OutDataTypeStr=single
  Gain3 : Gain  Gain=uT_to_gauss
  MAVLink Blank Message1 : uavmavlinklib/MAVLink Blank Message  dialectSource=Select from standard MAVLink dialects  dialect=common.xml  dialectCustom=common.xml  version=2  messageType=HIL_SENSOR  SystemID=2  ComponentID=51  SampleTime=SampleTime
  Multiply : Gain  Gain=SampleTime*1e6  OutDataTypeStr=Inherit: Inherit via back propagation
  Rate Transition : RateTransition
  Set this flag to indicate all flags are updated : Constant  Value=8191  OutDataTypeStr=Inherit: Inherit via back propagation  SampleTime=-1
  Temperature : Constant  Value=25  OutDataTypeStr=Inherit: Inherit via back propagation  SampleTime=-1
  HIL Sensor : Outport
  wires:
  Data Type Conversion2/1 -> Demux2/1
  Demux1/1 -> Bus Assignment1/6
  Mag/1 -> Gain3/1
  Demux1/3 -> Bus Assignment1/8
  Data Type Conversion1/1 -> Demux1/1
  Gyro/1 -> Data Type Conversion1/1
  Bus Assignment1/1 -> HIL Sensor/1
  Demux/3 -> Bus Assignment1/5
  Demux2/2 -> Bus Assignment1/10
  Demux2/3 -> Bus Assignment1/11
  Data Type Conversion5/1 -> Demux/1
  Demux/1 -> Bus Assignment1/3
  MAVLink Blank Message1/1 -> Bus Assignment1/1
  Demux2/1 -> Bus Assignment1/9
  Demux/2 -> Bus Assignment1/4
  Demux1/2 -> Bus Assignment1/7
  Acc/1 -> Data Type Conversion5/1
  Data Type Conversion3/1 -> Bus Assignment1/12
  Gain3/1 -> Data Type Conversion2/1
  Set this flag to indicate all flags are updated/1 -> Bus Assignment1/13
  Pressure/1 -> Gain2/1
  Clock/1 -> Rate Transition/1
  Rate Transition/1 -> Multiply/1
  Multiply/1 -> Bus Assignment1/2
  Gain2/1 -> Data Type Conversion3/1
  Temperature/1 -> Bus Assignment1/14

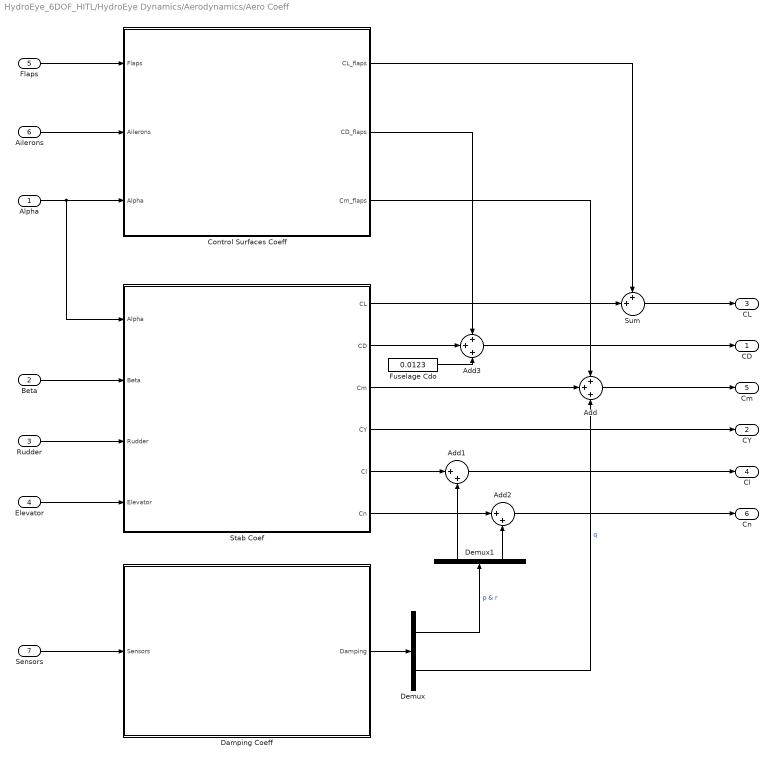
== system HydroEye_6DOF_HITL/HydroEye Dynamics/Aerodynamics/Aero Coeff ==
  Alpha : Inport
  Beta : Inport  Port=2
  Rudder : Inport  Port=3
  Elevator : Inport  Port=4
  Flaps : Inport  Port=5
  Ailerons : Inport  Port=6
  Sensors : Inport  Port=7
  Add : Sum  Inputs=+++
  Add1 : Sum  Inputs=|++
  Add2 : Sum  Inputs=|++
  Add3 : Sum  Inputs=+++
  Control Surfaces Coeff : Subsystem
  Damping Coeff : Subsystem
  Demux : Demux  Outputs=2
  Demux1 : Demux  Outputs=2
  Fuselage Cdo : Constant  Value=0.0123
  Stab Coef : Subsystem
  Sum : Sum  Inputs=++|
  CD : Outport
  CY : Outport  Port=2
  CL : Outport  Port=3
  Cl : Outport  Port=4
  Cm : Outport  Port=5
  Cn : Outport  Port=6
  wires:
  Alpha/1 -> Stab Coef/1(Alpha), Control Surfaces Coeff/3(Alpha)
  Beta/1 -> Stab Coef/2(Beta)
  Stab Coef/4(CY) -> CY/1
  Sensors/1 -> Damping Coeff/1(Sensors)
  Damping Coeff/1(Damping) -> Demux/1
  Stab Coef/3(Cm) -> Add/2
  Add/1 -> Cm/1
  Demux/2 -> Add/3  "q"
  Stab Coef/5(Cl) -> Add1/1
  Add1/1 -> Cl/1
  Add2/1 -> Cn/1
  Stab Coef/6(Cn) -> Add2/1
  Demux/1 -> Demux1/1  "p & r"
  Demux1/2 -> Add2/2
  Demux1/1 -> Add1/2
  Stab Coef/2(CD) -> Add3/2
  Add3/1 -> CD/1
  Fuselage Cdo/1 -> Add3/3
  Rudder/1 -> Stab Coef/3(Rudder)
  Elevator/1 -> Stab Coef/4(Elevator)
  Ailerons/1 -> Control Surfaces Coeff/2(Ailerons)
  Flaps/1 -> Control Surfaces Coeff/1(Flaps)
  Control Surfaces Coeff/2(CD_flaps) -> Add3/1
  Control Surfaces Coeff/3(Cm_flaps) -> Add/1
  Stab Coef/1(CL) -> Sum/2
  Control Surfaces Coeff/1(CL_flaps) -> Sum/1
  Sum/1 -> CL/1

== system HydroEye_6DOF_HITL/HydroEye Dynamics/Aerodynamics/Aerodynamic Coefficients ==
  Actuators : Inport  Unit=deg
  p,q,r : Inport  Port=2  Unit=rad/second
  V : Inport  Port=3  Unit=m/s
  Incid : Inport  Port=4  Unit=rad
  Actuator Increments : Subsystem
  Body Rate Damping : Subsystem
  Datum Coefficients : Subsystem
  Demux : Demux  Outputs=2
      settings: DisplayOption=none
  Sum1 : Sum  Inputs=+++  InputSameDT=on  SaturateOnIntegerOverflow=on  OutDataTypeStr=Inherit: Same as first input
  Coeff : Outport  InitialOutput=0  VectorParamsAs1DForOutWhenUnconnected=off
  wires:
  Demux/1 -> Datum Coefficients/1(Alpha), Actuator Increments/1(Alpha), Body Rate Damping/3(Alpha)
  p,q,r/1 -> Body Rate Damping/2(p,q,r)
  Incid/1 -> Demux/1
  Actuators/1 -> Actuator Increments/2("Actuator Deflections ")
  Sum1/1 -> Coeff/1
  Datum Coefficients/1(cl) -> Sum1/2
  Demux/2 -> Datum Coefficients/2(Beta)
  V/1 -> Body Rate Damping/1(V)
  Body Rate Damping/1(cl) -> Sum1/1
  Actuator Increments/1(cl) -> Sum1/3

== system HydroEye_6DOF_HITL/HydroEye Dynamics/Aerodynamics/Alpha,Beta,q ==
  Enviornmnet : Inport
  Sensors : Inport  Port=2
  Bus Selector : BusSelector  OutputSignals=rho
  Bus Selector1 : BusSelector  OutputSignals=Raw States.Vb
  Dynamic Pressure : aerolibasang/Dynamic Pressure
      settings: LibrarySourceBlock=|
      | aeroblk_lib_HL20/HL20
      | Airframe/Alpha,Beta,Mach/Dynamic Pressure
  "Incidence, Sideslip & Airspeed" : aerolibasang/Incidence, Sideslip, & Airspeed
      settings: LibrarySourceBlock=|
      | aeroblk_lib_HL20/HL20
      | Airframe/Alpha,Beta,Mach/Incidence, Sideslip
      | & Airspeed
  Mux : Mux  Inputs=2
  Incid : Outport  Unit=rad  VectorParamsAs1DForOutWhenUnconnected=off
  qbar : Outport  Port=2  Unit=Pa  InitialOutput=0  VectorParamsAs1DForOutWhenUnconnected=off
  wires:
  "Incidence, Sideslip & Airspeed"/1 -> Mux/1  "Alpha"
  Mux/1 -> Incid/1
  "Incidence, Sideslip & Airspeed"/2 -> Mux/2  "Beta"
  Dynamic Pressure/1 -> qbar/1
  Enviornmnet/1 -> Bus Selector/1
  Bus Selector/1 -> Dynamic Pressure/2  "<rho>"
  Sensors/1 -> Bus Selector1/1
  Bus Selector1/1 -> "Incidence, Sideslip & Airspeed"/1, Dynamic Pressure/1  "<Vb>"

== system HydroEye_6DOF_HITL/HydroEye Dynamics/Ground Model/Crash Detector ==
  F : Inport
  Compare To Constant : simulink/Logic and Bit Operations/Compare To Constant  relop=>  const=100  OutDataTypeStr=boolean
  Gain : Gain  Gain=1/mass/g
  norm1 : Subsystem
  crashFlag : Outport
  wires:
  F/1 -> norm1/1(F)
  norm1/1(Out1) -> Gain/1
  Compare To Constant/1 -> crashFlag/1
  Gain/1 -> Compare To Constant/1  "g's"

== system HydroEye_6DOF_HITL/HydroEye Dynamics/Ground Model/Friction Force ==
  V : Inport
  Fn : Inport  Port=2
  Product : Product
  Saturation : Saturate  UpperLimit=contact.translation.maxFriction  LowerLimit=-contact.translation.maxFriction
  Soft Coulomb Friction : Subsystem
  Unary Minus : UnaryMinus
  Friction : Outport
  wires:
  Fn/1 -> Product/2
  Soft Coulomb Friction/1(Out1) -> Product/1
  Product/1 -> Unary Minus/1
  V/1 -> Soft Coulomb Friction/1(In1)
  Unary Minus/1 -> Saturation/1
  Saturation/1 -> Friction/1

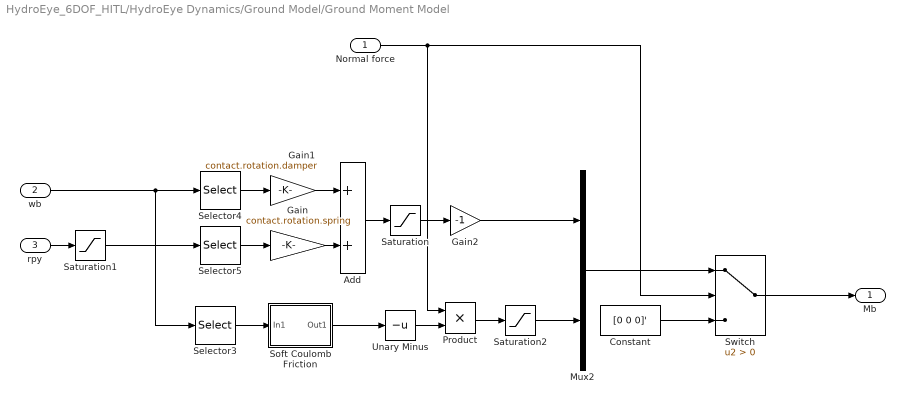
== system HydroEye_6DOF_HITL/HydroEye Dynamics/Ground Model/Ground Moment Model ==
  Normal force : Inport
  wb : Inport  Port=2
  rpy : Inport  Port=3
  Add : Sum
  Constant : Constant  Value=[0 0 0]'
  Gain : Gain  Gain=contact.rotation.spring
  Gain1 : Gain  Gain=contact.rotation.damper
  Gain2 : Gain  Gain=-1
  Mux2 : Mux  Inputs=2
  Product : Product
  Saturation : Saturate  UpperLimit=control.rotation.maxMoment  LowerLimit=-control.rotation.maxMoment
  Saturation1 : Saturate  UpperLimit=20*pi/180  LowerLimit=-20*pi/180
  Saturation2 : Saturate  UpperLimit=control.rotation.maxMoment  LowerLimit=-control.rotation.maxMoment
  Selector3 : Selector  InputPortWidth=3  IndexOptions=Index vector (dialog)  Indices=[3]  OutputSizes=1
  Selector4 : Selector  InputPortWidth=3  IndexOptions=Index vector (dialog)  Indices=[1, 2]  OutputSizes=1
  Selector5 : Selector  InputPortWidth=3  IndexOptions=Index vector (dialog)  Indices=[1, 2]  OutputSizes=1
  Soft Coulomb Friction : Subsystem
  Switch : Switch  Criteria=u2 > Threshold  SaturateOnIntegerOverflow=off  InputSameDT=off
  Unary Minus : UnaryMinus
  Mb : Outport
  wires:
  Gain2/1 -> Mux2/1
  Add/1 -> Saturation/1
  Gain/1 -> Add/2
  Saturation/1 -> Gain2/1
  Selector4/1 -> Gain1/1
  Gain1/1 -> Add/1
  Constant/1 -> Switch/3
  Selector5/1 -> Gain/1
  Switch/1 -> Mb/1
  Mux2/1 -> Switch/1
  Normal force/1 -> Product/1, Switch/2
  rpy/1 -> Saturation1/1
  Saturation1/1 -> Selector5/1
  wb/1 -> Selector4/1, Selector3/1
  Selector3/1 -> Soft Coulomb Friction/1(In1)
  Soft Coulomb Friction/1(Out1) -> Unary Minus/1
  Unary Minus/1 -> Product/2
  Product/1 -> Saturation2/1
  Saturation2/1 -> Mux2/2

== system HydroEye_6DOF_HITL/HydroEye Dynamics/Ground Model/Normal Force ==
  Vz : Inport
  Z : Inport  Port=2
  Add : Sum
  Constant : Constant  Value=0
  Damper Kp : Gain  Gain=-contact.translation.damper
  Saturation : Saturate  UpperLimit=contact.translation.maxNormal  LowerLimit=0
  Spring Kp : Gain  Gain=-contact.translation.spring
  Switch : Switch  Criteria=u2 > Threshold  SaturateOnIntegerOverflow=off  InputSameDT=off
  Unary Minus : UnaryMinus
  Unary Minus1 : UnaryMinus
  Normal : Outport
  wires:
  Constant/1 -> Switch/1
  Z/1 -> Unary Minus/1
  Switch/1 -> Saturation/1
  Damper Kp/1 -> Add/2
  Add/1 -> Switch/3
  Spring Kp/1 -> Add/1
  Vz/1 -> Unary Minus1/1
  Saturation/1 -> Normal/1
  Unary Minus/1 -> Spring Kp/1, Switch/2
  Unary Minus1/1 -> Damper Kp/1

== system HydroEye_6DOF_HITL/HydroEye Dynamics/Aerodynamics/Aero Coeff/Control Surfaces Coeff ==
  note: Ailerons
  note: Flaps
  Flaps : Inport
  Ailerons : Inport  Port=2
  Alpha : Inport  Port=3
  Lookup CD_flaps : Interpolation_n-D  Table=CD_flaps  InternalRulePriority=Speed
  Lookup CD_flaps1 : Interpolation_n-D  Table=Cm_flaps  InternalRulePriority=Speed
  Lookup CL_flaps : Interpolation_n-D  Table=CL_flaps  InternalRulePriority=Speed
  Prelookup : PreLookup  BreakpointsData=flaps  ExtrapMethod=Linear
  CL_flaps : Outport
  CD_flaps : Outport  Port=2
  Cm_flaps : Outport  Port=3
  wires:
  Prelookup/2 -> Lookup CD_flaps1/4, Lookup CD_flaps/4, Lookup CL_flaps/4
  Flaps/1 -> Prelookup/1
  Prelookup/1 -> Lookup CD_flaps1/3, Lookup CD_flaps/3, Lookup CL_flaps/3
  Lookup CD_flaps1/1 -> Cm_flaps/1
  Lookup CL_flaps/1 -> CL_flaps/1
  Lookup CD_flaps/1 -> CD_flaps/1
  Alpha/1 -> Lookup CD_flaps1/1, Lookup CD_flaps/1, Lookup CL_flaps/1, Lookup CD_flaps1/2, Lookup CD_flaps/2, Lookup CL_flaps/2

== system HydroEye_6DOF_HITL/HydroEye Dynamics/Aerodynamics/Aero Coeff/Damping Coeff ==
  Sensors : Inport
  Bus Selector : BusSelector  OutputSignals=Raw States.Angle Rate,Raw States.Vb
  Mux : Mux  Inputs=2
  p & r : Subsystem
  q : Subsystem
  Damping : Outport
  wires:
  Sensors/1 -> Bus Selector/1
  q/1(pitch rate damping) -> Mux/2
  Mux/1 -> Damping/1
  p & r/1(roll rate damping) -> Mux/1
  Bus Selector/1 -> p & r/1(<Angle Rate>), q/1(<Angle Rate>)  "<Angle Rate>"
  Bus Selector/2 -> q/2(<Vb>), p & r/2(<Vb>)  "<Vb>"

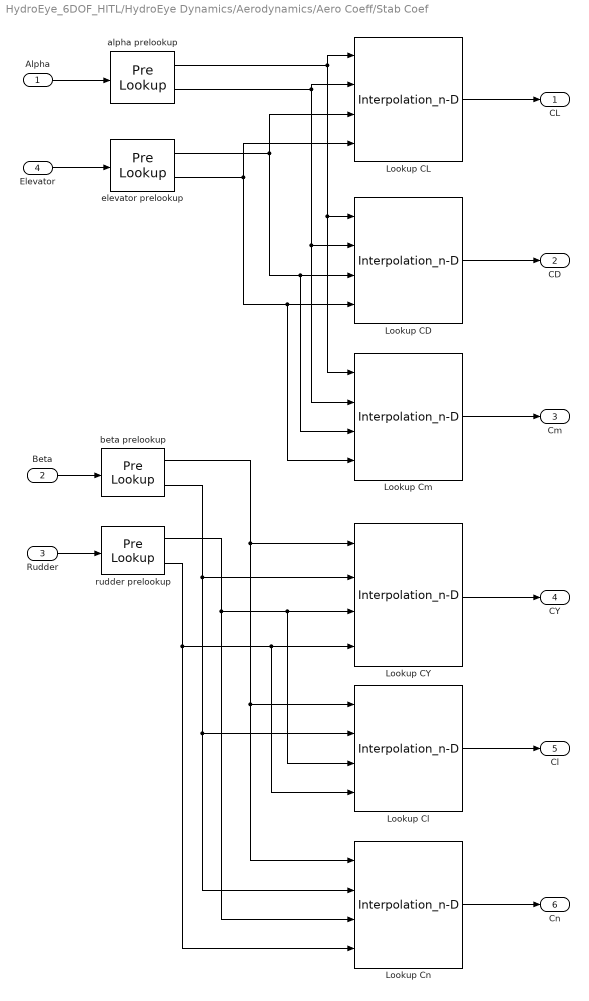
== system HydroEye_6DOF_HITL/HydroEye Dynamics/Aerodynamics/Aero Coeff/Stab Coef ==
  Alpha : Inport
  Beta : Inport  Port=2
  Rudder : Inport  Port=3
  Elevator : Inport  Port=4
  Lookup CD : Interpolation_n-D  Table=CDo_CD_elev  InternalRulePriority=Speed
  Lookup CL : Interpolation_n-D  Table=CLo_CL_elev  InternalRulePriority=Speed
  Lookup CY : Interpolation_n-D  Table=Cyo_Cy_rudder  InternalRulePriority=Speed
  Lookup Cl : Interpolation_n-D  Table=Clo_Cl_rudder  InternalRulePriority=Speed
  Lookup Cm : Interpolation_n-D  Table=Cmo_Cm_elev  InternalRulePriority=Speed
  Lookup Cn : Interpolation_n-D  Table=Cno_Cn_rudder  InternalRulePriority=Speed
  alpha prelookup : PreLookup  BreakpointsData=alpha  BeginIndexSearchUsingPreviousIndexResult=on  ExtrapMethod=Linear
  beta prelookup : PreLookup  BreakpointsData=beta  ExtrapMethod=Linear
  elevator prelookup : PreLookup  BreakpointsData=elevator  ExtrapMethod=Linear
  rudder prelookup : PreLookup  BreakpointsData=elevator  ExtrapMethod=Linear
  CL : Outport
  CD : Outport  Port=2
  Cm : Outport  Port=3
  CY : Outport  Port=4
  Cl : Outport  Port=5
  Cn : Outport  Port=6
  wires:
  beta prelookup/2 -> Lookup Cl/2, Lookup Cn/2, Lookup CY/2
  alpha prelookup/1 -> Lookup CL/1, Lookup Cm/1, Lookup CD/1
  beta prelookup/1 -> Lookup CY/1, Lookup Cl/1, Lookup Cn/1
  Lookup Cn/1 -> Cn/1
  Alpha/1 -> alpha prelookup/1
  alpha prelookup/2 -> Lookup Cm/2, Lookup CD/2, Lookup CL/2
  Lookup CL/1 -> CL/1
  Beta/1 -> beta prelookup/1
  Lookup Cm/1 -> Cm/1
  Rudder/1 -> rudder prelookup/1
  Lookup CY/1 -> CY/1
  Lookup Cl/1 -> Cl/1
  Lookup CD/1 -> CD/1
  Elevator/1 -> elevator prelookup/1
  elevator prelookup/1 -> Lookup CL/3, Lookup Cm/3, Lookup CD/3
  elevator prelookup/2 -> Lookup Cm/4, Lookup CD/4, Lookup CL/4
  rudder prelookup/1 -> Lookup Cn/3, Lookup Cl/3, Lookup CY/3
  rudder prelookup/2 -> Lookup Cn/4, Lookup Cl/4, Lookup CY/4
